simulink model "Copy_of_NolinearPMP"  (R2019b)
settings: Solver=ode14x  StartTime=0.0  StopTime=t_cyc(end)  FixedStep=0.01  RelTol=1e-3  EnableMultiTasking=on
values from neighbouring files (symbols this model uses):
  alph_cyc = [0 0 0 0 0 0 0 0 0 0 0 0 ... (6685 elements, 6685x1)]    [SUMOInfo.mat]
  distance_edge = [989.64 2422.29 340.79 475.79 617.54 348 731.29 242.71 400.49 162.3 1072.99 342.19 ... (42 elements, 42x1)]    [SUMOInfo.mat]    (also in msfun_EMS_PMP.m = block.DialogPrm(15).Data)
  ess_ro = block.DialogPrm(9).Data    [msfun_EMS_PMP.m]
  ess_soc = block.DialogPrm(7).Data    [msfun_EMS_PMP.m]
  ess_voc = block.DialogPrm(8).Data    [msfun_EMS_PMP.m]
  K = block.DialogPrm(12).Data    [msfun_EMS_PMP.m]
  meangrade = zeros(42,1)    [data_load.m]
  Np = block.DialogPrm(11).Data    [msfun_EMS_PMP.m]
  Ns = block.DialogPrm(10).Data    [msfun_EMS_PMP.m]
  p2 = block.DialogPrm(13).Data    [msfun_EMS_PMP.m]
  PM = block.DialogPrm(4).Data    [msfun_EMS_PMP.m]
  Qnom = block.DialogPrm(5).Data    [msfun_EMS_PMP.m]
  ratio = block.DialogPrm(3).Data    [msfun_EMS_PMP.m]
  regR = zeros(42,1)    [data_load.m]    (also in msfun_EMS_PMP.m = block.DialogPrm(6).Data)
  s = [0 1.19972903225 3.59869534029 7.19334975441 11.9718409783 17.9064273504 24.9452359727 33.006043999 41.9755365162 51.7163644674 62.0808345859 72.9273231974 ... (6685 elements, 6685x1)]    [SUMOInfo.mat]
  t_cyc = [1 2 3 4 5 6 7 8 9 10 11 12 ... (6685 elements, 6685x1)]    [SUMOInfo.mat]
  trafficspeed = block.DialogPrm(1).Data    [msfun_EMS_PMP.m]
  v_cyc = [0 4.31902451611 8.63627870893 12.9407558908 17.202568406 21.3645109397 25.3397110401 29.0189088948 32.2901730621 35.0669806241 37.3120924268 39.0473590013 ... (6685 elements, 6685x1)]    [SUMOInfo.mat]
undefined symbols (not defined in the file or in its folder): A_wind, Cd, Ce, delta1, delta2, eff_m, fuelrate, i0, Je, Jg, ki, kp, lambda_f, Ld, Lq, MaxFuelRate, meanspeed_record, motor_nt, nOpt, p, Pdmd_distribution, PgOpt, Qmax, R, r_wh, segmentID, Ta, veh_mass, x0
libraries: simulink x4, dsparch4 x1
settings Model: SimulationMode=accelerator  Creator=chenyaoqi  LastModifiedBy=Administrator
settings SolverCC: NumberNewtonIterations=2
settings DataIOCC: ReturnWorkspaceOutputs=off
settings OptimizationCC: LifeSpan=inf
settings DebuggingCC: SFUnexpectedBacktrackingDiag=warning  SFNoUnconditionalDefaultTransitionDiag=warning  ArithmeticOperatorsInVariantConditions=warning
settings SFSimCC: SimUseLocalCustomCode=off  CustomCodeUndefinedFunction=UseInterfaceOnly
settings RTWCC: RTWUseLocalCustomCode=off
settings CodeAppCC: StateflowObjectComments=on
settings GRTTargetCC: TargetLangStandard=C89/C90 (ANSI)  GeneratePreprocessorConditionals=Disable all
settings ConfigComp: CovMetricSettings=dw  CovHtmlReporting=on  CovSaveCumulativeToWorkspaceVar=on  CovSaveSingleToWorkspaceVar=on  CovExternalEMLEnable=off

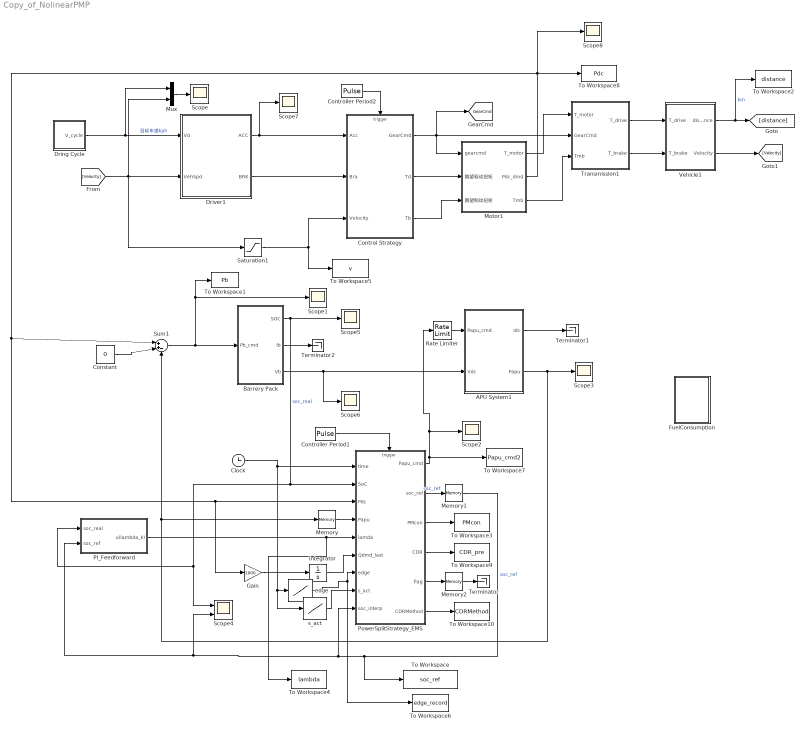
== system Copy_of_NolinearPMP ==
  APU System1 : Subsystem
  Barrery Pack : Subsystem
  Clock : Clock
  Constant : Constant  Value=0
  Control Strategy : Stateflow chart  TreatAsAtomicUnit=on
  Controller Period1 : DiscretePulseGenerator  PulseType=Time based  Period=1  PulseWidth=50
  Controller Period2 : DiscretePulseGenerator  PulseType=Time based  Period=0.1  PulseWidth=10
  Dring Cycle : Subsystem
  Driver1 : Subsystem
  FuelConsumption : Subsystem
  Gain : Gain  Gain=1000
  Integrator : Integrator
  Memory : Memory
  Memory1 : Memory
  Memory2 : Memory  InheritSampleTime=on
  Motor1 : Subsystem
  Mux : Mux  Inputs=2
  PI_Feedforward : Subsystem
  PowerSplitStrategy_EMS : Subsystem
  Rate Limiter : RateLimiter  RisingSlewLimit=8  FallingSlewLimit=-10
  Saturation1 : Saturate  UpperLimit=200  LowerLimit=0
  Scope{,1..3,5..8} (8 alike) : Scope
  Scope4 : Scope  NumInputPorts=2
  Sum1 : Sum  Inputs=|++-
  Terminator : Terminator
  Terminator1 : Terminator
  Terminator2 : Terminator
  To Workspace : ToWorkspace  VariableName=soc_ref  SampleTime=-1
  To Workspace1 : ToWorkspace  VariableName=Pb  SampleTime=-1
  To Workspace10 : ToWorkspace  VariableName=CDRMethod  SampleTime=-1
  To Workspace2 : ToWorkspace  VariableName=distance  SampleTime=-1
  To Workspace3 : ToWorkspace  VariableName=PMcon  SampleTime=-1
  To Workspace4 : ToWorkspace  VariableName=lambda  SampleTime=-1
  To Workspace5 : ToWorkspace  VariableName=v  SampleTime=-1
  To Workspace6 : ToWorkspace  VariableName=edge_record  SampleTime=-1
  To Workspace7 : ToWorkspace  VariableName=Papu_cmd2  SampleTime=-1
  To Workspace8 : ToWorkspace  VariableName=Pdc  SampleTime=-1
  To Workspace9 : ToWorkspace  VariableName=CDR_pre  SampleTime=-1
  Transmission1 : Subsystem
  Vehicle1 : Subsystem
  edge : Lookup  InputValues=t_cyc  Table=segmentID  LookUpMeth=Use Input Nearest
  s_act : Lookup  InputValues=t_cyc  Table=s
  tag scope: GearCmd=global
  wires:
  Barrery Pack/2(Ib) -> Terminator2/1
  Constant/1 -> Sum1/2
  PowerSplitStrategy_EMS/1(Papu_cmd) -> To Workspace7/1, Rate Limiter/1, Scope2/1
  Sum1/1 -> Barrery Pack/1(Pb_cmd), To Workspace1/1, Scope1/1
  APU System1/1(Idc) -> Terminator1/1
  Barrery Pack/3(Vb) -> Scope6/1, APU System1/2(Vdc)
  Rate Limiter/1 -> APU System1/1(Papu_cmd)
  Dring Cycle/1(V_cycle) -> Driver1/1(Vd), Mux/1  "目标车速kph"
  [Velocity] -> Driver1/2(VehSpd), Mux/2, Saturation1/1
  Saturation1/1 -> Control Strategy/3(Velocity), To Workspace5/1
  Barrery Pack/1(SOC) -> Scope5/1, Scope4/1, PI_Feedforward/1(soc_real), PowerSplitStrategy_EMS/2(SoC)  "soc_real"
  APU System1/2(Papu) -> Scope3/1, Sum1/3, Memory/1
  Controller Period1/1 -> PowerSplitStrategy_EMS/Trigger
  Mux/1 -> Scope/1
  Transmission1/1(T_drive) -> Vehicle1/1(T_drive)
  Motor1/1(T_motor) -> Transmission1/1(T_motor)
  Motor1/2(Pdc_dmd) -> Scope8/1, To Workspace8/1, Sum1/1, Gain/1, PowerSplitStrategy_EMS/3(Pdc)
  Controller Period2/1 -> Control Strategy/Trigger
  Control Strategy/1(GearCmd) -> [GearCmd], Transmission1/2(GearCmd), Motor1/1(gearcmd)
  Vehicle1/1(distance) -> [distance], To Workspace2/1  "km"
  Vehicle1/2(Velocity) -> [Velocity]
  Motor1/3(Tmb) -> Transmission1/3(Tmb)
  Control Strategy/2(Td) -> Motor1/2(期望驱动扭矩)
  Control Strategy/3(Tb) -> Motor1/3(期望制动扭矩)
  Transmission1/2(T_brake) -> Vehicle1/2(T_brake)
  Driver1/1(ACC) -> Scope7/1, Control Strategy/1(Acc)
  Driver1/2(BRK) -> Control Strategy/2(Bra)
  Memory/1 -> PowerSplitStrategy_EMS/4(Papu)
  Integrator/1 -> PowerSplitStrategy_EMS/6(Qdmd_last)
  edge/1 -> To Workspace6/1, PowerSplitStrategy_EMS/7(edge)
  Clock/1 -> PowerSplitStrategy_EMS/1(time), s_act/1, edge/1
  s_act/1 -> PowerSplitStrategy_EMS/8(s_act)
  Gain/1 -> Integrator/1
  Memory1/1 -> PI_Feedforward/2(soc_ref), Scope4/2, PowerSplitStrategy_EMS/9(soc_interp), To Workspace/1  "soc_ref"
  PowerSplitStrategy_EMS/3(PMcon) -> To Workspace3/1
  PowerSplitStrategy_EMS/4(CDR) -> To Workspace9/1
  PowerSplitStrategy_EMS/5(flag) -> Memory2/1
  Memory2/1 -> Terminator/1
  PowerSplitStrategy_EMS/6(CDRMethod) -> To Workspace10/1
  PI_Feedforward/1(u(lambda_k)) -> To Workspace4/1, PowerSplitStrategy_EMS/5(lamda)
  PowerSplitStrategy_EMS/2(soc_ref) -> Memory1/1  "soc_ref"

== system Copy_of_NolinearPMP/APU System1 ==
  Papu_cmd : Inport
  Vdc : Inport  Port=2
  "APU Optimal Operating LIne2 " : Lookup_n-D  NumberOfTableDimensions=1  BreakpointsForDimension1=PgOpt  Table=nOpt  InputSameDT=on
  Divide1 : Product  Inputs=/*
  Gain : Gain  Gain=9549
  Genset : Subsystem
  To Workspace1 : ToWorkspace  VariableName=Papu  SampleTime=-1
  Idc : Outport
  Papu : Outport  Port=2
  tag scope: Papu=global
  wires:
  Papu_cmd/1 -> Gain/1, "APU Optimal Operating LIne2 "/1
  Gain/1 -> Divide1/2
  Genset/1(Ig) -> Idc/1
  Genset/2(Papu) -> To Workspace1/1, Papu/1, [Papu]
  Vdc/1 -> Genset/2(Vdc)  "pack电压"
  "APU Optimal Operating LIne2 "/1 -> Divide1/1, Genset/3(omega_cmd)  "期望转速rpm"
  Divide1/1 -> Genset/1(T_cmd)  "期望扭矩"

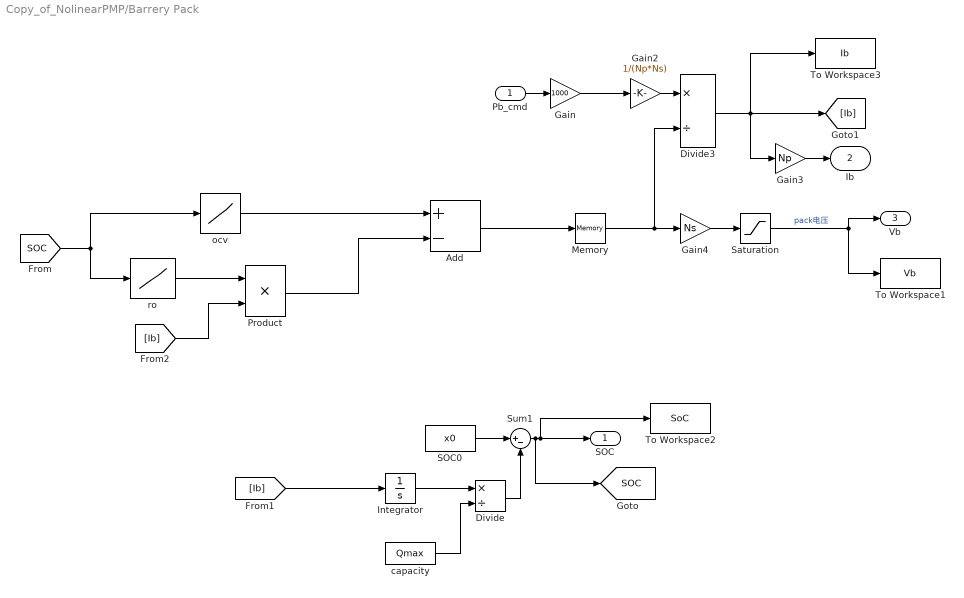
== system Copy_of_NolinearPMP/Barrery Pack ==
  Pb_cmd : Inport
  Add : Sum  Inputs=+-
  Divide : Product  Inputs=*/
  Divide3 : Product  Inputs=*/
  Gain : Gain  Gain=1000
  Gain2 : Gain  Gain=1/(Np*Ns)
  Gain3 : Gain  Gain=Np
  Gain4 : Gain  Gain=Ns
  Integrator : Integrator
  Memory : Memory  InitialCondition=4
  Product : Product
  SOC0 : Constant  Value=x0
  Saturation : Saturate  UpperLimit=453.6  LowerLimit=302.4
  Sum1 : Sum  Inputs=|+-
  To Workspace1 : ToWorkspace  VariableName=Vb  SampleTime=-1
  To Workspace2 : ToWorkspace  VariableName=SoC  SampleTime=-1
  To Workspace3 : ToWorkspace  VariableName=Ib  SampleTime=-1
  capacity : Constant  Value=Qmax
  ocv : Lookup_n-D  NumberOfTableDimensions=1  BreakpointsForDimension1=ess_soc  Table=ess_voc  InternalRulePriority=Speed  RndMeth=Simplest  InputSameDT=on
  ro : Lookup_n-D  NumberOfTableDimensions=1  BreakpointsForDimension1=ess_soc  Table=ess_ro  InternalRulePriority=Speed  RndMeth=Simplest  InputSameDT=on
  SOC : Outport
  Ib : Outport  Port=2
  Vb : Outport  Port=3
  tag scope: SOC=global
  wires:
  capacity/1 -> Divide/2
  Divide/1 -> Sum1/2
  SOC0/1 -> Sum1/1
  Sum1/1 -> [SOC], SOC/1, To Workspace2/1
  Integrator/1 -> Divide/1
  Pb_cmd/1 -> Gain/1
  Gain/1 -> Gain2/1
  Divide3/1 -> To Workspace3/1, Gain3/1, [Ib]
  Memory/1 -> Divide3/2, Gain4/1
  Gain2/1 -> Divide3/1
  [SOC] -> ocv/1, ro/1
  Gain3/1 -> Ib/1
  Gain4/1 -> Saturation/1
  Saturation/1 -> To Workspace1/1, Vb/1  "pack电压"
  ro/1 -> Product/1
  [Ib] -> Product/2
  Add/1 -> Memory/1
  ocv/1 -> Add/1
  Product/1 -> Add/2
  [Ib] -> Integrator/1

== system Copy_of_NolinearPMP/Dring Cycle ==
  Clock : Clock
  To Workspace1 : ToWorkspace  VariableName=time  SampleTime=-1
  cyc : Lookup  InputValues=t_cyc  Table=v_cyc  LookUpMeth=Interpolation-Use End Values
  V_cycle : Outport
  wires:
  Clock/1 -> cyc/1, To Workspace1/1
  cyc/1 -> V_cycle/1  "kph"

== system Copy_of_NolinearPMP/Driver1 ==
  Vd : Inport
  VehSpd : Inport  Port=2
  Clock : Clock
  Driver : Subsystem
  Mux1 : Mux  Inputs=2
  alph_cyc : Lookup  InputValues=t_cyc  Table=alph_cyc
  黄色-模型车速、蓝色-实际车速 : Scope
  ACC : Outport
  BRK : Outport  Port=2
  wires:
  VehSpd/1 -> Driver/2(VelFdbk), Mux1/2  "模型仿真车速"
  Vd/1 -> Mux1/1, Driver/1(VelRef)
  Mux1/1 -> 黄色-模型车速、蓝色-实际车速/1
  Driver/1(AccelCmd) -> ACC/1
  Driver/2(BrkCmd) -> BRK/1
  alph_cyc/1 -> Driver/3(Grade)
  Clock/1 -> alph_cyc/1

== system Copy_of_NolinearPMP/FuelConsumption ==
  Constant : Constant  Value=0
  FuelRate : Fcn  Expr=Ce(1)+Ce(2)*u(1)+Ce(3)*u(2)+Ce(4)*u(1)*u(1)+Ce(5)*u(1)*u(2)+Ce(6)*u(2)*u(2)+Ce(7)*u(1)*u(1)*u(1)+Ce(8)*u(1)*u(1)*u(2)+Ce(9)*u(1)*u(2)*u(2)+Ce(10)*u(2)*u(2)*u(2)
  Gain : Gain  Gain=30/pi
  Integrator : Integrator
  Mux : Mux  Inputs=2
  Switch : Switch
  To Workspace : ToWorkspace  VariableName=CumulativeFC  SampleTime=-1
  To Workspace1 : ToWorkspace  VariableName=FC_instant  SampleTime=-1
  wires:
  [Te] -> Mux/2
  Mux/1 -> FuelRate/1
  [omega_e] -> Gain/1
  Gain/1 -> Mux/1  "rpm"
  Integrator/1 -> To Workspace/1
  FuelRate/1 -> Switch/2, Switch/1
  Switch/1 -> Integrator/1, To Workspace1/1
  Constant/1 -> Switch/3

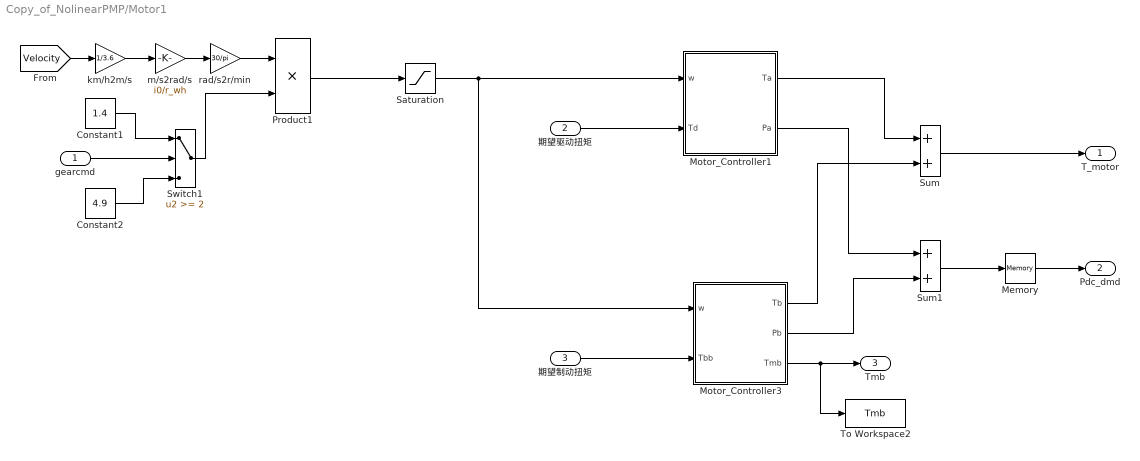
== system Copy_of_NolinearPMP/Motor1 ==
  gearcmd : Inport
  期望驱动扭矩 : Inport  Port=2
  期望制动扭矩 : Inport  Port=3
  Constant1 : Constant  Value=1.4
  Constant2 : Constant  Value=4.9
  Memory : Memory  InheritSampleTime=on
  Motor_Controller1 : Subsystem
  Motor_Controller3 : Subsystem
  Product1 : Product  RndMeth=Zero
  Saturation : Saturate  UpperLimit=4200  LowerLimit=0  ZeroCross=off
  Sum : Sum
  Sum1 : Sum
  Switch1 : Switch  Threshold=2  ZeroCross=off
  To Workspace2 : ToWorkspace  VariableName=Tmb  SampleTime=-1
      settings: Decimation=100
  km/h2m/s : Gain  Gain=1/3.6
  m/s2rad/s : Gain  Gain=i0/r_wh
  rad/s2r/min : Gain  Gain=30/pi
  T_motor : Outport
  Pdc_dmd : Outport  Port=2
  Tmb : Outport  Port=3
  wires:
  Sum1/1 -> Memory/1
  km/h2m/s/1 -> m/s2rad/s/1
  [Velocity] -> km/h2m/s/1
  gearcmd/1 -> Switch1/2
  Constant1/1 -> Switch1/1
  Constant2/1 -> Switch1/3
  Switch1/1 -> Product1/2
  Sum/1 -> T_motor/1
  m/s2rad/s/1 -> rad/s2r/min/1
  rad/s2r/min/1 -> Product1/1
  Product1/1 -> Saturation/1
  Memory/1 -> Pdc_dmd/1
  Saturation/1 -> Motor_Controller1/1(w), Motor_Controller3/1(w)
  期望驱动扭矩/1 -> Motor_Controller1/2(Td)
  期望制动扭矩/1 -> Motor_Controller3/2(Tbb)
  Motor_Controller3/3(Tmb) -> To Workspace2/1, Tmb/1
  Motor_Controller3/2(Pb) -> Sum1/2
  Motor_Controller1/2(Pa) -> Sum1/1
  Motor_Controller1/1(Ta) -> Sum/1
  Motor_Controller3/1(Tb) -> Sum/2

== system Copy_of_NolinearPMP/PI_Feedforward ==
  soc_real : Inport
  soc_ref : Inport  Port=2
  Add : Sum  Inputs=+-
  Analog Filter Design : dsparch4/Analog Filter Design  Commented=on  method=Butterworth  filttype=Lowpass  N=1  Wlo=0.5  Whi=80  Rp=2  Rs=40
  PID Controller : simulink/Continuous/PID Controller  Controller=PI  Form=Parallel  TimeDomain=Continuous-time  SampleTime=-1  IntegratorMethod=Forward Euler  FilterMethod=Forward Euler  ControllerParametersSource=internal  P=kp  I=ki  D=0  UseFilter=on  N=100  TunerSelectOption=Transfer Function Based (PID Tuner App)  InitialConditionSource=internal  InitialConditionForIntegrator=-13066.5  InitialConditionForFilter=0  DifferentiatorICPrevScaledInput=0  ExternalReset=none  TrackingMode=off  Kt=1  LimitOutput=off  UpperSaturationLimit=inf  LowerSaturationLimit=-inf  LinearizeAsGain=on  AntiWindupMode=none  Kb=1  POutMin=[]  POutMax=[]  IOutMin=[]  IOutMax=[]  DOutMin=[]  DOutMax=[]  NOutMin=[]  NOutMax=[]  SumOutMin=[]  SumOutMax=[]  SaturationOutMin=[]  SaturationOutMax=[]  PParamMin=[]  PParamMax=[]  IParamMin=[]  IParamMax=[]  DParamMin=[]  DParamMax=[]  NParamMin=[]  NParamMax=[]  KbParamMin=[]  KbParamMax=[]  KtParamMin=[]  KtParamMax=[]  KbOutMin=[]  KbOutMax=[]  KtOutMin=[]  KtOutMax=[]  IntegratorOutMin=[]  IntegratorOutMax=[]  FilterOutMin=[]  FilterOutMax=[]  SumI1OutMin=[]  SumI1OutMax=[]  SumI2OutMin=[]  SumI2OutMax=[]  SumI3OutMin=[]  SumI3OutMax=[]  SumI4OutMin=[]  SumI4OutMax=[]  SumDOutMin=[]  SumDOutMax=[]  DifferentiatorOutMin=[]  DifferentiatorOutMax=[]  FilterDiffOutCoefMin=[]  FilterDiffOutCoefMax=[]  ReciprocalOutMin=[]  ReciprocalOutMax=[]  SumDenOutMin=[]  SumDenOutMax=[]  SumNumOutMin=[]  SumNumOutMax=[]  DivideOutMin=[]  DivideOutMax=[]  IntegratorContinuousStateAttributes=''  IntegratorStateMustResolveToSignalObject=off  IntegratorRTWStateStorageClass=Auto  FilterContinuousStateAttributes=''  FilterStateMustResolveToSignalObject=off  FilterRTWStateStorageClass=Auto  ParallelPVariant=InternalParameters  IdealPVariant=Disabled  IVariant=InternalParameters  DVariant=Disabled  IntegratorVariant=Continuous  SatVariant=Disabled  AWVariant=Passthrough  PCopyVariant=Disabled  TRVariant=Disabled  FdbkBlocksVariant=Forward  IdealPFdbkVariant=Disabled  SatFdbkVariant=Disabled  DerivativeFilterVariant=Disabled  NVariant=Disabled  NCopyVariant=Disabled_SignalSpec  FilterICVariant=Disabled  IntegratorICVariant=InternalICs  ExternalResetVariant=Disabled  TRSumVariant=Passthrough  SumFdbkVariant=Disabled  SumVariant=Sum_PI
  u(lambda_k) : Outport  InitialOutput=-13060  VectorParamsAs1DForOutWhenUnconnected=off
  wires:
  soc_real/1 -> Add/1
  soc_ref/1 -> Add/2
  PID Controller/1 -> u(lambda_k)/1  "delta_u"
  Add/1 -> PID Controller/1  "e(k)"

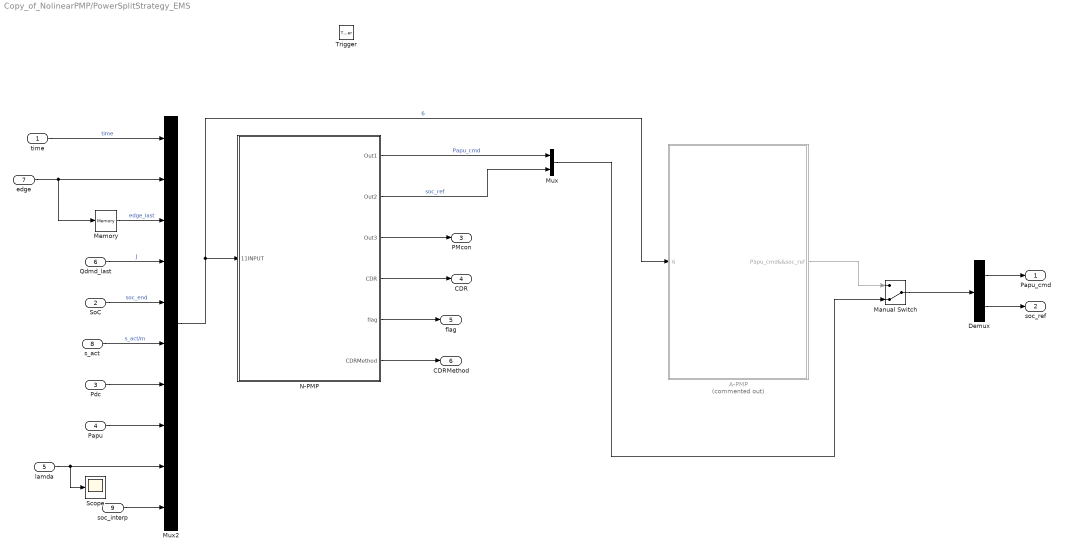
== system Copy_of_NolinearPMP/PowerSplitStrategy_EMS ==
  time : Inport
  SoC : Inport  Port=2
  Pdc : Inport  Port=3
  Papu : Inport  Port=4
  lamda : Inport  Port=5
  Qdmd_last : Inport  Port=6
  edge : Inport  Port=7
  s_act : Inport  Port=8
  soc_interp : Inport  Port=9
  Trigger : TriggerPort  VariantControl=Variant  PortDimensions=1
  A-PMP : Subsystem  Commented=on
  Demux : Demux  Outputs=2
  Manual Switch : ManualSwitch  CurrentSetting=0
  Memory : Memory  InitialCondition=1  InheritSampleTime=on
  Mux : Mux  Inputs=2
  Mux2 : Mux  Inputs=10
  N-PMP : Subsystem
  Scope : Scope
  Papu_cmd : Outport
  soc_ref : Outport  Port=2
  PMcon : Outport  Port=3  VectorParamsAs1DForOutWhenUnconnected=off
  CDR : Outport  Port=4  VectorParamsAs1DForOutWhenUnconnected=off
  flag : Outport  Port=5  VectorParamsAs1DForOutWhenUnconnected=off
  CDRMethod : Outport  Port=6  VectorParamsAs1DForOutWhenUnconnected=off
  wires:
  Mux2/1 -> A-PMP/1(6), N-PMP/1(11INPUT)  "6"
  A-PMP/1(Papu_cmd&&soc_ref) -> Manual Switch/1
  Mux/1 -> Manual Switch/2
  Manual Switch/1 -> Demux/1
  Demux/1 -> Papu_cmd/1
  Demux/2 -> soc_ref/1
  lamda/1 -> Scope/1, Mux2/9
  N-PMP/1(Out1) -> Mux/1  "Papu_cmd"
  N-PMP/2(Out2) -> Mux/2  "soc_ref"
  time/1 -> Mux2/1  "time"
  edge/1 -> Mux2/2, Memory/1
  Memory/1 -> Mux2/3  "edge_last"
  Pdc/1 -> Mux2/7
  SoC/1 -> Mux2/5  "soc_end"
  s_act/1 -> Mux2/6  "s_act/m"
  Papu/1 -> Mux2/8
  Qdmd_last/1 -> Mux2/4  "J"
  N-PMP/3(Out3) -> PMcon/1
  N-PMP/4(CDR) -> CDR/1
  soc_interp/1 -> Mux2/10
  N-PMP/5(flag) -> flag/1
  N-PMP/6(CDRMethod) -> CDRMethod/1

== system Copy_of_NolinearPMP/Transmission1 ==
  T_motor : Inport
  GearCmd : Inport  Port=2
  Tmb : Inport  Port=3
  Gain : Gain  Gain=0.95
  Gain1 : Gain  Gain=0.95
  Lookup Table : Lookup  InputValues=[1,2]  Table=[4.9,1.4]
  Product : Product  RndMeth=Zero
  Product1 : Product  RndMeth=Zero
  T_drive : Outport
  T_brake : Outport  Port=2
  wires:
  GearCmd/1 -> Lookup Table/1
  T_motor/1 -> Product/1
  Lookup Table/1 -> Product/2, Product1/2
  Gain/1 -> T_drive/1
  Product/1 -> Gain/1
  Tmb/1 -> Product1/1
  Gain1/1 -> T_brake/1
  Product1/1 -> Gain1/1

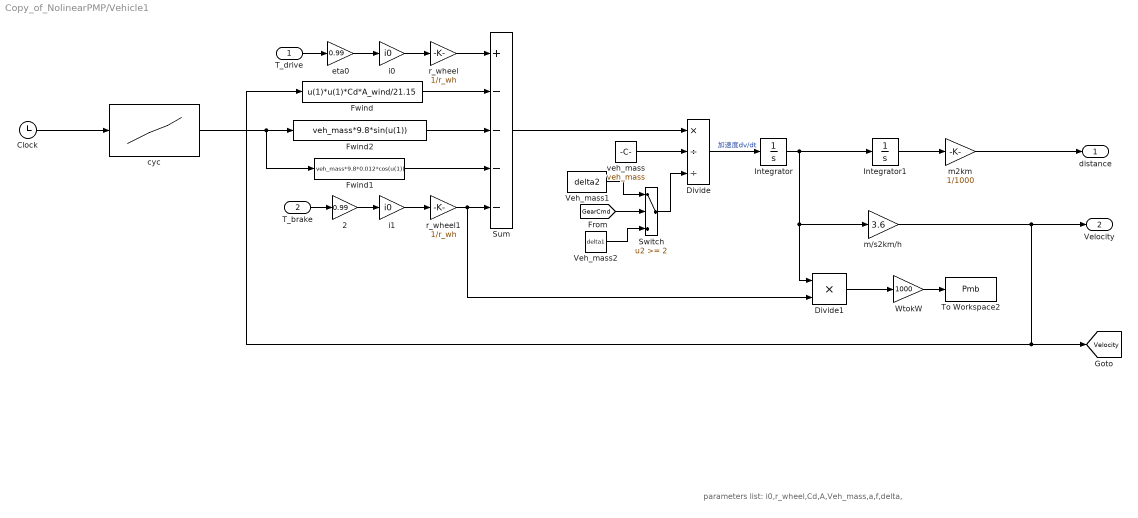
== system Copy_of_NolinearPMP/Vehicle1 ==
  note: parameters list: i0,r_wheel,Cd,A,Veh_mass,a,f,delta,
  T_drive : Inport
  T_brake : Inport  Port=2
  2 : Gain  Gain=0.99
  Clock : Clock
  Divide : Product  Inputs=*//
  Divide1 : Product  Inputs=**
  Fwind : Fcn  Expr=u(1)*u(1)*Cd*A_wind/21.15
  Fwind1 : Fcn  Expr=veh_mass*9.8*0.012*cos(u(1))
  Fwind2 : Fcn  Expr=veh_mass*9.8*sin(u(1))
  Integrator : Integrator  LimitOutput=on  UpperSaturationLimit=100  LowerSaturationLimit=0
  Integrator1 : Integrator
  Sum : Sum  Inputs=+----
  Switch : Switch  Threshold=2  ZeroCross=off
  To Workspace2 : ToWorkspace  VariableName=Pmb  SampleTime=-1
  Veh_mass1 : Constant  Value=delta2
  Veh_mass2 : Constant  Value=delta1
  WtokW : Gain  Gain=1000
  cyc : Lookup  InputValues=t_cyc  Table=alph_cyc
  eta0 : Gain  Gain=0.99
  i0 : Gain  Gain=i0
  i1 : Gain  Gain=i0
  m/s2km/h : Gain  Gain=3.6
  m2km : Gain  Gain=1/1000
  r_wheel : Gain  Gain=1/r_wh
  r_wheel1 : Gain  Gain=1/r_wh
  veh_mass : Constant  Value=veh_mass
  distance : Outport
  Velocity : Outport  Port=2
  tag scope: Velocity=global
  wires:
  Fwind1/1 -> Sum/4
  Fwind2/1 -> Sum/3
  Fwind/1 -> Sum/2
  r_wheel/1 -> Sum/1
  Sum/1 -> Divide/1
  veh_mass/1 -> Divide/2
  Divide/1 -> Integrator/1  "加速度dv/dt"
  Integrator/1 -> Divide1/1, m/s2km/h/1, Integrator1/1
  m/s2km/h/1 -> Velocity/1, Fwind/1, [Velocity]
  Integrator1/1 -> m2km/1
  m2km/1 -> distance/1
  Switch/1 -> Divide/3
  Veh_mass1/1 -> Switch/1
  [GearCmd] -> Switch/2
  Veh_mass2/1 -> Switch/3
  cyc/1 -> Fwind1/1, Fwind2/1
  Clock/1 -> cyc/1
  i1/1 -> r_wheel1/1
  T_brake/1 -> 2/1
  2/1 -> i1/1
  r_wheel1/1 -> Divide1/2, Sum/5
  Divide1/1 -> WtokW/1
  WtokW/1 -> To Workspace2/1
  T_drive/1 -> eta0/1
  eta0/1 -> i0/1
  i0/1 -> r_wheel/1

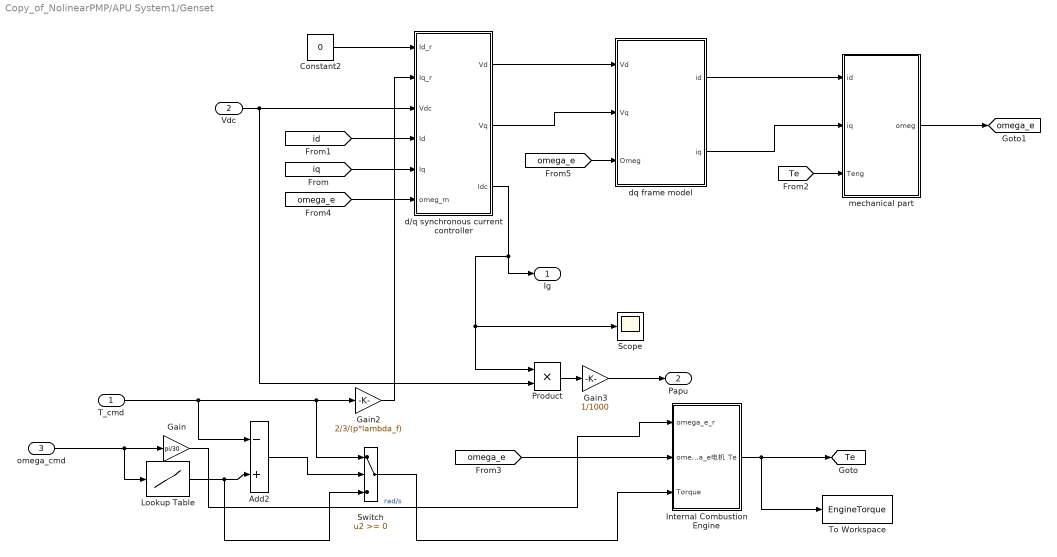
== system Copy_of_NolinearPMP/APU System1/Genset ==
  T_cmd : Inport
  Vdc : Inport  Port=2
  omega_cmd : Inport  Port=3
  Add2 : Sum  Inputs=-+
  Constant2 : Constant  Value=0
  Gain : Gain  Gain=pi/30
  Gain2 : Gain  Gain=2/3/(p*lambda_f)
  Gain3 : Gain  Gain=1/1000
  Internal Combustion Engine : Subsystem
  Lookup Table : Lookup  InputValues=[850,1000,1250,1500,1750,2000,2250,2500,2750,3000,3250,3500,3750,4000]  Table=[195,195,195,195.9,244.1,270.2,272.7,269.1,266.6,261.5,257.7,242.9,229.9,221.4]
  Product : Product  RndMeth=Zero
  Scope : Scope
  Switch : Switch
  To Workspace : ToWorkspace  VariableName=EngineTorque  SampleTime=-1
  d/q synchronous current controller : Subsystem
  "dq frame model " : Subsystem
  mechanical part : Subsystem
  Ig : Outport
  Papu : Outport  Port=2
  tag scope: Te=global, omega_e=global
  wires:
  mechanical part/1(omeg) -> [omega_e]
  "dq frame model "/1(id) -> mechanical part/1(id)
  "dq frame model "/2(iq) -> mechanical part/2(iq)
  [Te] -> mechanical part/3(Teng)
  [id] -> d/q synchronous current controller/4(Id)
  [iq] -> d/q synchronous current controller/5(Iq)
  [omega_e] -> Internal Combustion Engine/2(omega_e电机)
  [omega_e] -> d/q synchronous current controller/6(omeg_m)
  [omega_e] -> "dq frame model "/3(Omeg)
  Constant2/1 -> d/q synchronous current controller/1(Id_r)
  Vdc/1 -> Product/2, d/q synchronous current controller/3(Vdc)
  d/q synchronous current controller/3(Idc) -> Scope/1, Product/1, Ig/1
  Product/1 -> Gain3/1
  Internal Combustion Engine/1(Te) -> [Te], To Workspace/1
  omega_cmd/1 -> Lookup Table/1, Gain/1
  Gain2/1 -> d/q synchronous current controller/2(Iq_r)
  d/q synchronous current controller/1(Vd) -> "dq frame model "/1(Vd)
  d/q synchronous current controller/2(Vq) -> "dq frame model "/2(Vq)
  T_cmd/1 -> Add2/1, Gain2/1, Switch/1
  Lookup Table/1 -> Add2/2, Switch/3
  Add2/1 -> Switch/2
  Switch/1 -> Internal Combustion Engine/3(Torque)
  Gain/1 -> Internal Combustion Engine/1(omega_e_r)  "rad/s"
  Gain3/1 -> Papu/1

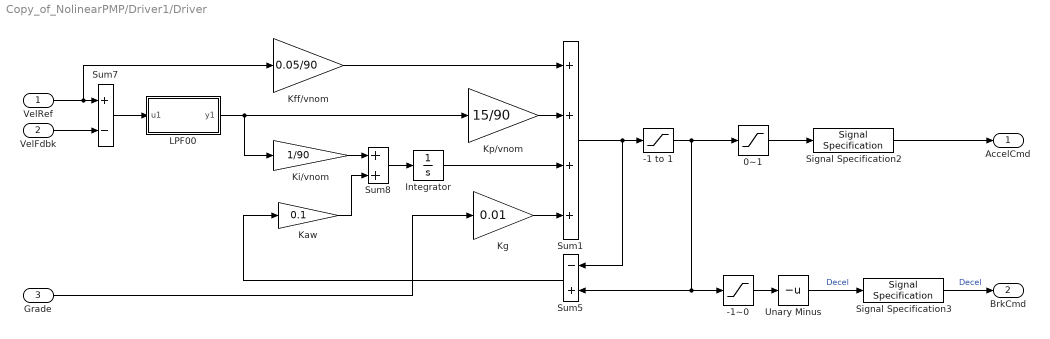
== system Copy_of_NolinearPMP/Driver1/Driver ==
  VelRef : Inport
  VelFdbk : Inport  Port=2
  Grade : Inport  Port=3
  "-1 to 1 " : Saturate  UpperLimit=1  LowerLimit=-1
  -1~0 : Saturate  UpperLimit=0  LowerLimit=-1  ZeroCross=off
  0~1 : Saturate  UpperLimit=1  LowerLimit=0  ZeroCross=off
  Integrator : Integrator  LimitOutput=on  UpperSaturationLimit=1  LowerSaturationLimit=-1
  Kaw : Gain  Gain=0.1  SaturateOnIntegerOverflow=on  OutDataTypeStr=Inherit: Same as input  ParamDataTypeStr=Inherit: Same as input
  Kff/vnom : Gain  Gain=0.05/90  SaturateOnIntegerOverflow=on  OutDataTypeStr=Inherit: Same as input  ParamDataTypeStr=Inherit: Same as input
  Kg : Gain  Gain=0.01  SaturateOnIntegerOverflow=on  OutDataTypeStr=Inherit: Same as input  ParamDataTypeStr=Inherit: Same as input
  Ki/vnom : Gain  Gain=1/90  SaturateOnIntegerOverflow=on  OutDataTypeStr=Inherit: Same as input  ParamDataTypeStr=Inherit: Same as input
  Kp/vnom : Gain  Gain=15/90  SaturateOnIntegerOverflow=on  OutDataTypeStr=Inherit: Same as input  ParamDataTypeStr=Inherit: Same as input
  LPF00 : Subsystem
  Signal Specification2 : SignalSpecification
  Signal Specification3 : SignalSpecification
  Sum1 : Sum  Inputs=++++  SaturateOnIntegerOverflow=on  InputSameDT=on  OutDataTypeStr=Inherit: Same as first input
  Sum5 : Sum  Inputs=-+  SaturateOnIntegerOverflow=on  InputSameDT=on  OutDataTypeStr=Inherit: Same as first input
  Sum7 : Sum  Inputs=+-  SaturateOnIntegerOverflow=on  InputSameDT=on  OutDataTypeStr=Inherit: Same as first input
  Sum8 : Sum  SaturateOnIntegerOverflow=on  InputSameDT=on  OutDataTypeStr=Inherit: Same as first input
  Unary Minus : UnaryMinus
  AccelCmd : Outport  InitialOutput=0
  BrkCmd : Outport  Port=2  InitialOutput=0
  wires:
  Sum7/1 -> LPF00/1(u1)
  0~1/1 -> Signal Specification2/1
  Sum1/1 -> "-1 to 1 "/1, Sum5/1
  LPF00/1(y1) -> Kp/vnom/1, Ki/vnom/1
  -1~0/1 -> Unary Minus/1
  VelFdbk/1 -> Sum7/2
  Kg/1 -> Sum1/4
  Grade/1 -> Kg/1
  Sum8/1 -> Integrator/1
  Kaw/1 -> Sum8/2
  Kp/vnom/1 -> Sum1/2
  "-1 to 1 "/1 -> 0~1/1, -1~0/1, Sum5/2
  VelRef/1 -> Sum7/1, Kff/vnom/1
  Unary Minus/1 -> Signal Specification3/1  "Decel"
  Kff/vnom/1 -> Sum1/1
  Integrator/1 -> Sum1/3
  Sum5/1 -> Kaw/1
  Ki/vnom/1 -> Sum8/1
  Signal Specification3/1 -> BrkCmd/1  "Decel"
  Signal Specification2/1 -> AccelCmd/1

== system Copy_of_NolinearPMP/Motor1/Motor_Controller1 ==
  w : Inport
  Td : Inport  Port=2
  2-D Lookup Table : Lookup_n-D  BreakpointsForDimension1=0:500:4500  BreakpointsForDimension2=-850:50:850  Table=eff_m  InternalRulePriority=Speed  RndMeth=Simplest  InputSameDT=on
  Divide : Product  Inputs=*/
  Gain2 : Gain  Gain=1/9549
  Gain3 : Gain
  Lookup Table (3-D) : Lookup_n-D  BreakpointsForDimension1=[500,1000,1500,2000,2500,3000,3500,4000,4200]  BreakpointsForDimension2=[0,800,1600,2400,3200,4000,4800,5600,6400,7200,8000]  BreakpointsForDimension3=[425,445]  Table=Ta  InputSameDT=on
  Product : Product  RndMeth=Zero
  Saturation : Saturate  UpperLimit=1  LowerLimit=0.1
  Ta : Outport
  Pa : Outport  Port=2
  wires:
  Divide/1 -> Pa/1
  Td/1 -> Lookup Table (3-D)/2
  Lookup Table (3-D)/1 -> Product/1, Gain3/1
  Product/1 -> Gain2/1
  w/1 -> Lookup Table (3-D)/1, Product/2, 2-D Lookup Table/1
  Saturation/1 -> Divide/2
  2-D Lookup Table/1 -> Saturation/1
  Gain2/1 -> Divide/1
  Gain3/1 -> 2-D Lookup Table/2, Ta/1

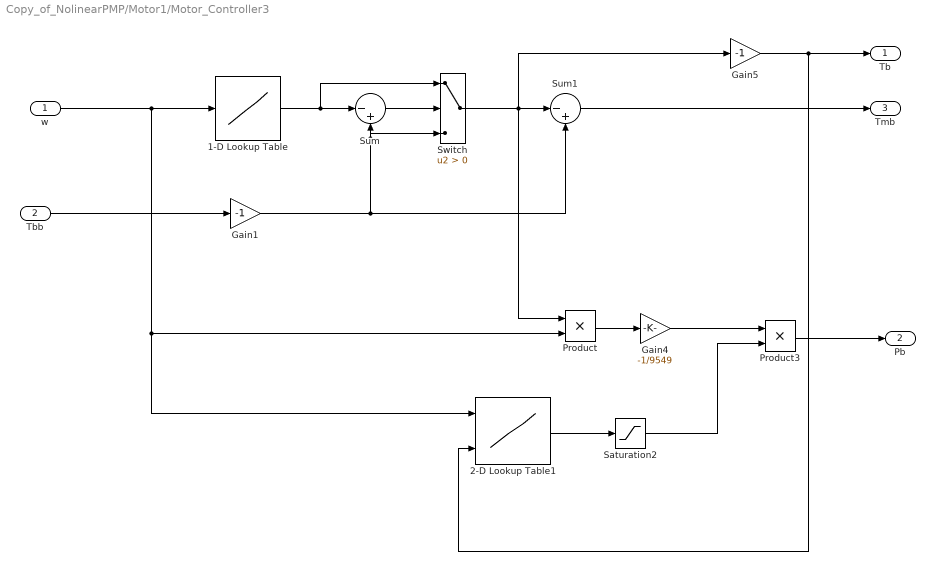
== system Copy_of_NolinearPMP/Motor1/Motor_Controller3 ==
  w : Inport
  Tbb : Inport  Port=2
  1-D Lookup Table : Lookup_n-D  NumberOfTableDimensions=1  BreakpointsForDimension1=motor_nt(:,1)  Table=motor_nt(:,2)*0.6  InternalRulePriority=Speed  RndMeth=Simplest  InputSameDT=on
  2-D Lookup Table1 : Lookup_n-D  BreakpointsForDimension1=0:500:4500  BreakpointsForDimension2=-850:50:850  Table=eff_m  InternalRulePriority=Speed  RndMeth=Simplest  InputSameDT=on
  Gain1 : Gain  Gain=-1
  Gain4 : Gain  Gain=-1/9549
  Gain5 : Gain  Gain=-1
  Product : Product  RndMeth=Zero
  Product3 : Product  RndMeth=Zero
  Saturation2 : Saturate  UpperLimit=1  LowerLimit=0.1
  Sum : Sum  Inputs=|-+
  Sum1 : Sum  Inputs=|-+
  Switch : Switch  Criteria=u2 > Threshold
  Tb : Outport
  Pb : Outport  Port=2
  Tmb : Outport  Port=3
  wires:
  Product/1 -> Gain4/1
  2-D Lookup Table1/1 -> Saturation2/1
  Gain4/1 -> Product3/1
  Tbb/1 -> Gain1/1
  Product3/1 -> Pb/1
  w/1 -> 2-D Lookup Table1/1, Product/2, 1-D Lookup Table/1
  Gain5/1 -> 2-D Lookup Table1/2, Tb/1
  Sum/1 -> Switch/2
  Switch/1 -> Gain5/1, Product/1, Sum1/1
  1-D Lookup Table/1 -> Switch/1, Sum/1
  Gain1/1 -> Sum1/2, Switch/3, Sum/2
  Sum1/1 -> Tmb/1
  Saturation2/1 -> Product3/2

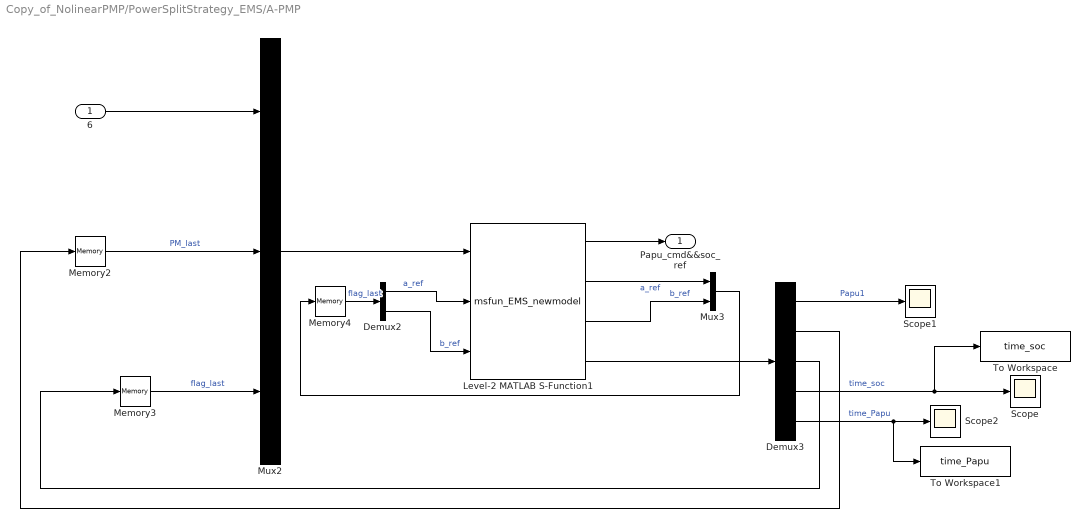
== system Copy_of_NolinearPMP/PowerSplitStrategy_EMS/A-PMP ==
  6 : Inport
  Demux2 : Demux  Outputs=2
  Demux3 : Demux  Outputs=5
  Level-2 MATLAB S-Function1 : M-S-Function  FunctionName=msfun_EMS_newmodel  Parameters=alph_cyc,s,t_cyc,v_cyc,trafficspeed,ess_soc,ess_voc,ess_ro,Np,Ns,Qmax,p2
  Memory2 : Memory  InheritSampleTime=on
  Memory3 : Memory  InheritSampleTime=on
  Memory4 : Memory  InheritSampleTime=on
  Mux2 : Mux  Inputs=3
  Mux3 : Mux  Inputs=2
  Scope : Scope
  Scope1 : Scope
  Scope2 : Scope
  To Workspace : ToWorkspace  VariableName=time_soc  SampleTime=-1
  To Workspace1 : ToWorkspace  VariableName=time_Papu  SampleTime=-1
  Papu_cmd&&soc_ref : Outport
  wires:
  Level-2 MATLAB S-Function1/4 -> Demux3/1
  Memory2/1 -> Mux2/2  "PM_last"
  Demux3/3 -> Memory3/1
  Demux3/2 -> Memory2/1
  Level-2 MATLAB S-Function1/3 -> Mux3/2  "b_ref"
  Level-2 MATLAB S-Function1/2 -> Mux3/1  "a_ref"
  Memory4/1 -> Demux2/1  "flag_last"
  Mux3/1 -> Memory4/1
  Mux2/1 -> Level-2 MATLAB S-Function1/1
  Demux3/1 -> Scope1/1  "Papu1"
  Demux2/1 -> Level-2 MATLAB S-Function1/2  "a_ref"
  Demux2/2 -> Level-2 MATLAB S-Function1/3  "b_ref"
  Memory3/1 -> Mux2/3  "flag_last"
  Level-2 MATLAB S-Function1/1 -> Papu_cmd&&soc_ref/1
  6/1 -> Mux2/1
  Demux3/4 -> To Workspace/1, Scope/1  "time_soc"
  Demux3/5 -> To Workspace1/1, Scope2/1  "time_Papu"

== system Copy_of_NolinearPMP/PowerSplitStrategy_EMS/N-PMP ==
  11INPUT : Inport
  Demux1 : Demux  Outputs=2
  Demux2 : Demux
  Level-2 MATLAB S-Function : M-S-Function  FunctionName=msfun_EMS_PMP  Parameters=meanspeed_record,meangrade,ratio,PM,Qnom,regR,ess_soc,ess_voc,ess_ro,Ns,Np,K,p2,Pdmd_distribution,distance_edge
  Memory1 : Memory  InheritSampleTime=on
  Mux1 : Mux  Inputs=2
  Out1 : Outport
  Out2 : Outport  Port=2
  Out3 : Outport  Port=3  VectorParamsAs1DForOutWhenUnconnected=off
  CDR : Outport  Port=4  VectorParamsAs1DForOutWhenUnconnected=off
  flag : Outport  Port=5  VectorParamsAs1DForOutWhenUnconnected=off
  CDRMethod : Outport  Port=6  VectorParamsAs1DForOutWhenUnconnected=off
  wires:
  Demux1/1 -> Level-2 MATLAB S-Function/2  "s_ref_last"
  Level-2 MATLAB S-Function/2 -> Mux1/1  "s_ref"
  Demux1/2 -> Level-2 MATLAB S-Function/3  "SOC_ref_last"
  Mux1/1 -> Memory1/1
  Memory1/1 -> Demux1/1
  Level-2 MATLAB S-Function/3 -> Mux1/2  "SOC_ref"
  Level-2 MATLAB S-Function/1 -> Demux2/1
  11INPUT/1 -> Level-2 MATLAB S-Function/1
  Demux2/2 -> Out2/1  "soc_ref"
  Demux2/1 -> Out1/1  "Papu_cmd"
  Demux2/3 -> Out3/1  "PMcon"
  Level-2 MATLAB S-Function/4 -> CDR/1
  Demux2/4 -> flag/1
  Level-2 MATLAB S-Function/5 -> CDRMethod/1

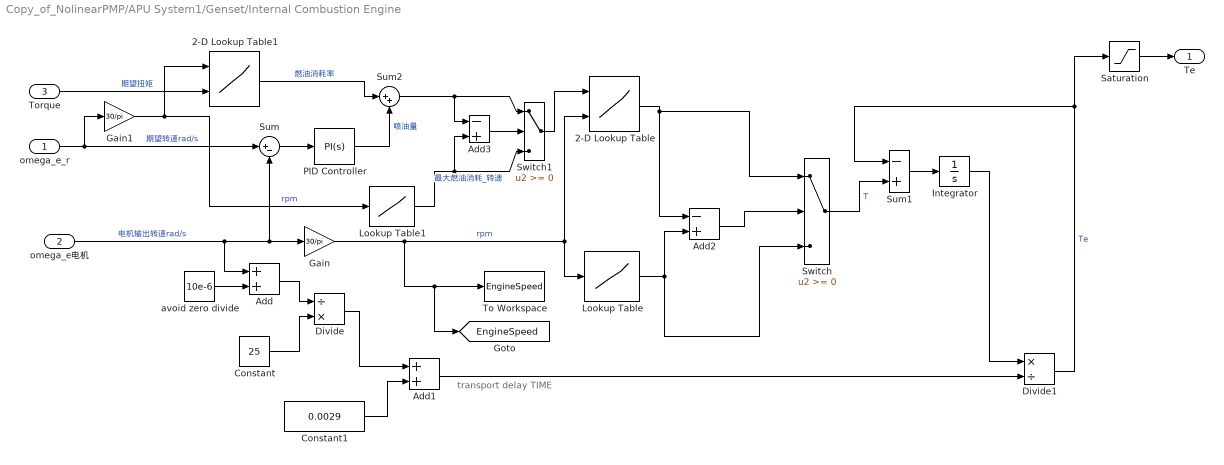
== system Copy_of_NolinearPMP/APU System1/Genset/Internal Combustion Engine ==
  note: transport delay TIME
  omega_e_r : Inport
  omega_e电机 : Inport  Port=2
  Torque : Inport  Port=3
  2-D Lookup Table : Lookup_n-D  BreakpointsForDimension1=0:0.1:5  BreakpointsForDimension2=1000:250:3000  Table=BrakeTorque'  InputSameDT=on
  2-D Lookup Table1 : Lookup_n-D  BreakpointsForDimension1=1000:250:3000  BreakpointsForDimension2=0:5:275  Table=fuelrate  InputSameDT=on
  Add : Sum
  Add1 : Sum
  Add2 : Sum  Inputs=-+
  Add3 : Sum  Inputs=-+
  Constant : Constant  Value=25
  Constant1 : Constant  Value=0.0029
  Divide : Product  Inputs=/*
  Divide1 : Product  Inputs=*/
  Gain : Gain  Gain=30/pi
  Gain1 : Gain  Gain=30/pi
  Integrator : Integrator
  Lookup Table : Lookup  InputValues=[850,1000,1250,1500,1750,2000,2250,2500,2750,3000,3250,3500,3750,4000]  Table=[195,195,195,195.9,244.1,270.2,272.7,269.1,266.6,261.5,257.7,242.9,229.9,221.4]
  Lookup Table1 : Lookup  InputValues=[1000,1250,1500,1750,2000,2250,2500,2750,3000]  Table=MaxFuelRate
  PID Controller : simulink/Continuous/PID Controller  Controller=PI  Form=Parallel  TimeDomain=Continuous-time  SampleTime=-1  IntegratorMethod=Forward Euler  FilterMethod=Forward Euler  ControllerParametersSource=internal  P=0.1  I=0.2  D=0  UseFilter=on  N=100  TunerSelectOption=Transfer Function Based (PID Tuner App)  InitialConditionSource=internal  InitialConditionForIntegrator=0  InitialConditionForFilter=0  DifferentiatorICPrevScaledInput=0  ExternalReset=none  TrackingMode=off  Kt=1  LimitOutput=off  UpperSaturationLimit=inf  LowerSaturationLimit=-inf  LinearizeAsGain=on  AntiWindupMode=none  Kb=1  POutMin=[]  POutMax=[]  IOutMin=[]  IOutMax=[]  DOutMin=[]  DOutMax=[]  NOutMin=[]  NOutMax=[]  SumOutMin=[]  SumOutMax=[]  SaturationOutMin=[]  SaturationOutMax=[]  PParamMin=[]  PParamMax=[]  IParamMin=[]  IParamMax=[]  DParamMin=[]  DParamMax=[]  NParamMin=[]  NParamMax=[]  KbParamMin=[]  KbParamMax=[]  KtParamMin=[]  KtParamMax=[]  KbOutMin=[]  KbOutMax=[]  KtOutMin=[]  KtOutMax=[]  IntegratorOutMin=[]  IntegratorOutMax=[]  FilterOutMin=[]  FilterOutMax=[]  SumI1OutMin=[]  SumI1OutMax=[]  SumI2OutMin=[]  SumI2OutMax=[]  SumI3OutMin=[]  SumI3OutMax=[]  SumI4OutMin=[]  SumI4OutMax=[]  SumDOutMin=[]  SumDOutMax=[]  DifferentiatorOutMin=[]  DifferentiatorOutMax=[]  FilterDiffOutCoefMin=[]  FilterDiffOutCoefMax=[]  ReciprocalOutMin=[]  ReciprocalOutMax=[]  SumDenOutMin=[]  SumDenOutMax=[]  SumNumOutMin=[]  SumNumOutMax=[]  DivideOutMin=[]  DivideOutMax=[]  IntegratorContinuousStateAttributes=''  IntegratorStateMustResolveToSignalObject=off  IntegratorRTWStateStorageClass=Auto  FilterContinuousStateAttributes=''  FilterStateMustResolveToSignalObject=off  FilterRTWStateStorageClass=Auto  ParallelPVariant=InternalParameters  IdealPVariant=Disabled  IVariant=InternalParameters  DVariant=Disabled  IntegratorVariant=Continuous  SatVariant=Disabled  AWVariant=Passthrough  PCopyVariant=Disabled  TRVariant=Disabled  FdbkBlocksVariant=Forward  IdealPFdbkVariant=Disabled  SatFdbkVariant=Disabled  DerivativeFilterVariant=Disabled  NVariant=Disabled  NCopyVariant=Disabled_SignalSpec  FilterICVariant=Disabled  IntegratorICVariant=InternalICs  ExternalResetVariant=Disabled  TRSumVariant=Passthrough  SumFdbkVariant=Disabled  SumVariant=Sum_PI
  Saturation : Saturate  UpperLimit=280  LowerLimit=0  LinearizeAsGain=off
  Sum : Sum  Inputs=|+-
  Sum1 : Sum  Inputs=-+
  Sum2 : Sum  Inputs=|++
  Switch : Switch
  Switch1 : Switch
  To Workspace : ToWorkspace  VariableName=EngineSpeed  SampleTime=-1
  avoid zero divide : Constant  Value=10e-6
  Te : Outport
  tag scope: EngineSpeed=global
  wires:
  omega_e电机/1 -> Add/1, Sum/2, Gain/1  "电机输出转速rad/s"
  Sum/1 -> PID Controller/1
  avoid zero divide/1 -> Add/2
  Constant/1 -> Divide/2
  Add/1 -> Divide/1
  Divide/1 -> Add1/1
  Constant1/1 -> Add1/2
  Add1/1 -> Divide1/2
  Integrator/1 -> Divide1/1
  Sum1/1 -> Integrator/1
  2-D Lookup Table/1 -> Add2/1, Switch/1
  Lookup Table/1 -> Add2/2, Switch/3
  Divide1/1 -> Sum1/1, Saturation/1  "Te"
  omega_e_r/1 -> Gain1/1, Sum/1  "期望转速rad/s"
  Gain/1 -> Lookup Table/1, 2-D Lookup Table/2, To Workspace/1, [EngineSpeed]  "rpm"
  Add2/1 -> Switch/2
  Switch/1 -> Sum1/2  "T"
  2-D Lookup Table1/1 -> Sum2/1  "燃油消耗率"
  PID Controller/1 -> Sum2/2  "喷油量"
  Sum2/1 -> Add3/1, Switch1/1
  Torque/1 -> 2-D Lookup Table1/2  "期望扭矩"
  Gain1/1 -> 2-D Lookup Table1/1, Lookup Table1/1  "rpm"
  Lookup Table1/1 -> Add3/2, Switch1/3  "最大燃油消耗_转速"
  Add3/1 -> Switch1/2
  Switch1/1 -> 2-D Lookup Table/1
  Saturation/1 -> Te/1

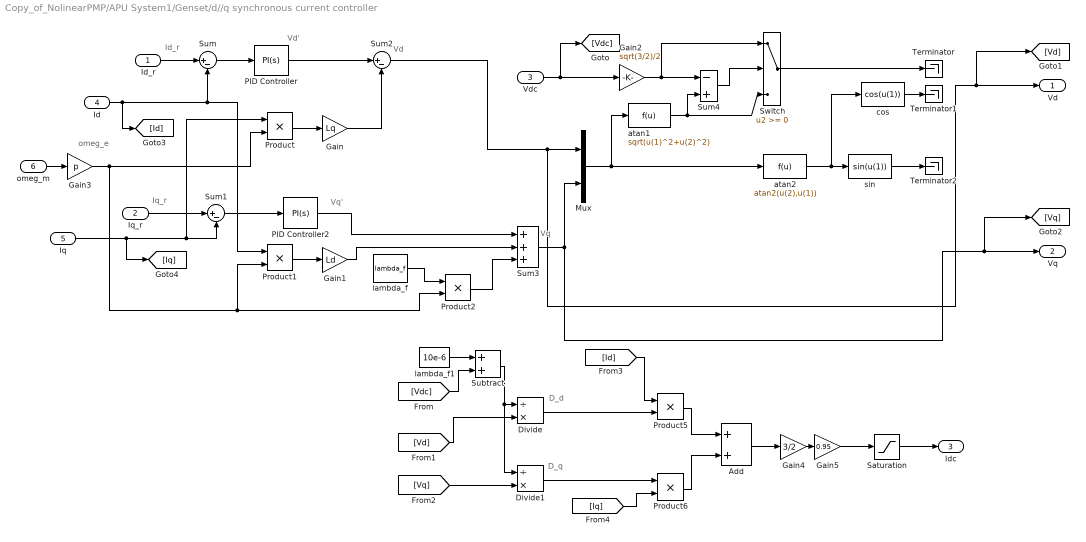
== system Copy_of_NolinearPMP/APU System1/Genset/d//q synchronous current controller ==
  note: Id_r
  note: Iq_r
  note: Vd'
  note: Vq'
  note: Vd
  note: Vq
  note: omeg_e
  note: D_d
  note: D_q
  Id_r : Inport
  Iq_r : Inport  Port=2
  Vdc : Inport  Port=3
  Id : Inport  Port=4
  Iq : Inport  Port=5
  omeg_m : Inport  Port=6
  Add : Sum
  Divide : Product  Inputs=/*
  Divide1 : Product  Inputs=/*
  Gain : Gain  Gain=Lq
  Gain1 : Gain  Gain=Ld
  Gain2 : Gain  Gain=sqrt(3/2)/2
  Gain3 : Gain  Gain=p
  Gain4 : Gain  Gain=3/2
  Gain5 : Gain  Gain=0.95
  Mux : Mux  Inputs=2
  PID Controller : simulink/Continuous/PID Controller  Controller=PI  Form=Parallel  TimeDomain=Continuous-time  SampleTime=-1  IntegratorMethod=Forward Euler  FilterMethod=Forward Euler  ControllerParametersSource=internal  P=0.003  I=0.01  D=0  UseFilter=on  N=100  TunerSelectOption=Transfer Function Based (PID Tuner App)  InitialConditionSource=internal  InitialConditionForIntegrator=0  InitialConditionForFilter=0  DifferentiatorICPrevScaledInput=0  ExternalReset=none  TrackingMode=off  Kt=1  LimitOutput=off  UpperSaturationLimit=inf  LowerSaturationLimit=-inf  LinearizeAsGain=on  AntiWindupMode=none  Kb=1  POutMin=[]  POutMax=[]  IOutMin=[]  IOutMax=[]  DOutMin=[]  DOutMax=[]  NOutMin=[]  NOutMax=[]  SumOutMin=[]  SumOutMax=[]  SaturationOutMin=[]  SaturationOutMax=[]  PParamMin=[]  PParamMax=[]  IParamMin=[]  IParamMax=[]  DParamMin=[]  DParamMax=[]  NParamMin=[]  NParamMax=[]  KbParamMin=[]  KbParamMax=[]  KtParamMin=[]  KtParamMax=[]  KbOutMin=[]  KbOutMax=[]  KtOutMin=[]  KtOutMax=[]  IntegratorOutMin=[]  IntegratorOutMax=[]  FilterOutMin=[]  FilterOutMax=[]  SumI1OutMin=[]  SumI1OutMax=[]  SumI2OutMin=[]  SumI2OutMax=[]  SumI3OutMin=[]  SumI3OutMax=[]  SumI4OutMin=[]  SumI4OutMax=[]  SumDOutMin=[]  SumDOutMax=[]  DifferentiatorOutMin=[]  DifferentiatorOutMax=[]  FilterDiffOutCoefMin=[]  FilterDiffOutCoefMax=[]  ReciprocalOutMin=[]  ReciprocalOutMax=[]  SumDenOutMin=[]  SumDenOutMax=[]  SumNumOutMin=[]  SumNumOutMax=[]  DivideOutMin=[]  DivideOutMax=[]  IntegratorContinuousStateAttributes=''  IntegratorStateMustResolveToSignalObject=off  IntegratorRTWStateStorageClass=Auto  FilterContinuousStateAttributes=''  FilterStateMustResolveToSignalObject=off  FilterRTWStateStorageClass=Auto  ParallelPVariant=InternalParameters  IdealPVariant=Disabled  IVariant=InternalParameters  DVariant=Disabled  IntegratorVariant=Continuous  SatVariant=Disabled  AWVariant=Passthrough  PCopyVariant=Disabled  TRVariant=Disabled  FdbkBlocksVariant=Forward  IdealPFdbkVariant=Disabled  SatFdbkVariant=Disabled  DerivativeFilterVariant=Disabled  NVariant=Disabled  NCopyVariant=Disabled_SignalSpec  FilterICVariant=Disabled  IntegratorICVariant=InternalICs  ExternalResetVariant=Disabled  TRSumVariant=Passthrough  SumFdbkVariant=Disabled  SumVariant=Sum_PI
  PID Controller2 : simulink/Continuous/PID Controller  Controller=PI  Form=Parallel  TimeDomain=Continuous-time  SampleTime=-1  IntegratorMethod=Forward Euler  FilterMethod=Forward Euler  ControllerParametersSource=internal  P=0.3  I=0.3  D=0  UseFilter=on  N=100  TunerSelectOption=Transfer Function Based (PID Tuner App)  InitialConditionSource=internal  InitialConditionForIntegrator=0  InitialConditionForFilter=0  DifferentiatorICPrevScaledInput=0  ExternalReset=none  TrackingMode=off  Kt=1  LimitOutput=off  UpperSaturationLimit=inf  LowerSaturationLimit=-inf  LinearizeAsGain=on  AntiWindupMode=none  Kb=1  POutMin=[]  POutMax=[]  IOutMin=[]  IOutMax=[]  DOutMin=[]  DOutMax=[]  NOutMin=[]  NOutMax=[]  SumOutMin=[]  SumOutMax=[]  SaturationOutMin=[]  SaturationOutMax=[]  PParamMin=[]  PParamMax=[]  IParamMin=[]  IParamMax=[]  DParamMin=[]  DParamMax=[]  NParamMin=[]  NParamMax=[]  KbParamMin=[]  KbParamMax=[]  KtParamMin=[]  KtParamMax=[]  KbOutMin=[]  KbOutMax=[]  KtOutMin=[]  KtOutMax=[]  IntegratorOutMin=[]  IntegratorOutMax=[]  FilterOutMin=[]  FilterOutMax=[]  SumI1OutMin=[]  SumI1OutMax=[]  SumI2OutMin=[]  SumI2OutMax=[]  SumI3OutMin=[]  SumI3OutMax=[]  SumI4OutMin=[]  SumI4OutMax=[]  SumDOutMin=[]  SumDOutMax=[]  DifferentiatorOutMin=[]  DifferentiatorOutMax=[]  FilterDiffOutCoefMin=[]  FilterDiffOutCoefMax=[]  ReciprocalOutMin=[]  ReciprocalOutMax=[]  SumDenOutMin=[]  SumDenOutMax=[]  SumNumOutMin=[]  SumNumOutMax=[]  DivideOutMin=[]  DivideOutMax=[]  IntegratorContinuousStateAttributes=''  IntegratorStateMustResolveToSignalObject=off  IntegratorRTWStateStorageClass=Auto  FilterContinuousStateAttributes=''  FilterStateMustResolveToSignalObject=off  FilterRTWStateStorageClass=Auto  ParallelPVariant=InternalParameters  IdealPVariant=Disabled  IVariant=InternalParameters  DVariant=Disabled  IntegratorVariant=Continuous  SatVariant=Disabled  AWVariant=Passthrough  PCopyVariant=Disabled  TRVariant=Disabled  FdbkBlocksVariant=Forward  IdealPFdbkVariant=Disabled  SatFdbkVariant=Disabled  DerivativeFilterVariant=Disabled  NVariant=Disabled  NCopyVariant=Disabled_SignalSpec  FilterICVariant=Disabled  IntegratorICVariant=InternalICs  ExternalResetVariant=Disabled  TRSumVariant=Passthrough  SumFdbkVariant=Disabled  SumVariant=Sum_PI
  Product{,1..2,5..6} (5 alike) : Product  RndMeth=Zero
  Saturation : Saturate  UpperLimit=180  LowerLimit=0
  Subtract : Sum
  Sum : Sum  Inputs=|+-
  Sum1 : Sum  Inputs=|+-
  Sum2 : Sum  Inputs=|+-
  Sum3 : Sum  Inputs=+++
  Sum4 : Sum  Inputs=-+
  Switch : Switch
  Terminator : Terminator
  Terminator1 : Terminator
  Terminator2 : Terminator
  atan1 : Fcn  Expr=sqrt(u(1)^2+u(2)^2)
  atan2 : Fcn  Expr=atan2(u(2),u(1))
  cos : Fcn  Expr=cos(u(1))
  lambda_f : Constant  Value=lambda_f
  lambda_f1 : Constant  Value=10e-6
  sin : Fcn  Expr=sin(u(1))
  Vd : Outport
  Vq : Outport  Port=2
  Idc : Outport  Port=3
  wires:
  Id_r/1 -> Sum/1
  Id/1 -> Sum/2, Product1/1, [Id]
  Sum/1 -> PID Controller/1
  Iq_r/1 -> Sum1/1
  Sum1/1 -> PID Controller2/1
  PID Controller/1 -> Sum2/1
  Product/1 -> Gain/1
  Gain/1 -> Sum2/2
  Sum2/1 -> Mux/1, Vd/1, [Vd]
  Product1/1 -> Gain1/1
  Gain1/1 -> Sum3/2
  Product2/1 -> Sum3/3
  lambda_f/1 -> Product2/1
  Sum3/1 -> Mux/2, Vq/1, [Vq]
  Mux/1 -> atan1/1, atan2/1
  atan2/1 -> cos/1, sin/1
  cos/1 -> Terminator1/1
  sin/1 -> Terminator2/1
  Iq/1 -> Sum1/2, Product/1, [Iq]
  Gain3/1 -> Product/2, Product1/2, Product2/2
  omeg_m/1 -> Gain3/1
  Vdc/1 -> [Vdc], Gain2/1
  atan1/1 -> Sum4/2, Switch/3
  Sum4/1 -> Switch/2
  Switch/1 -> Terminator/1
  PID Controller2/1 -> Sum3/1
  [Vdc] -> Subtract/2
  [Vd] -> Divide/2
  [Vq] -> Divide1/2
  [Id] -> Product5/1
  Divide/1 -> Product5/2
  Divide1/1 -> Product6/1
  [Iq] -> Product6/2
  Product5/1 -> Add/1
  Product6/1 -> Add/2
  Add/1 -> Gain4/1
  Gain4/1 -> Gain5/1
  lambda_f1/1 -> Subtract/1
  Subtract/1 -> Divide1/1, Divide/1
  Saturation/1 -> Idc/1
  Gain5/1 -> Saturation/1
  Gain2/1 -> Sum4/1, Switch/1

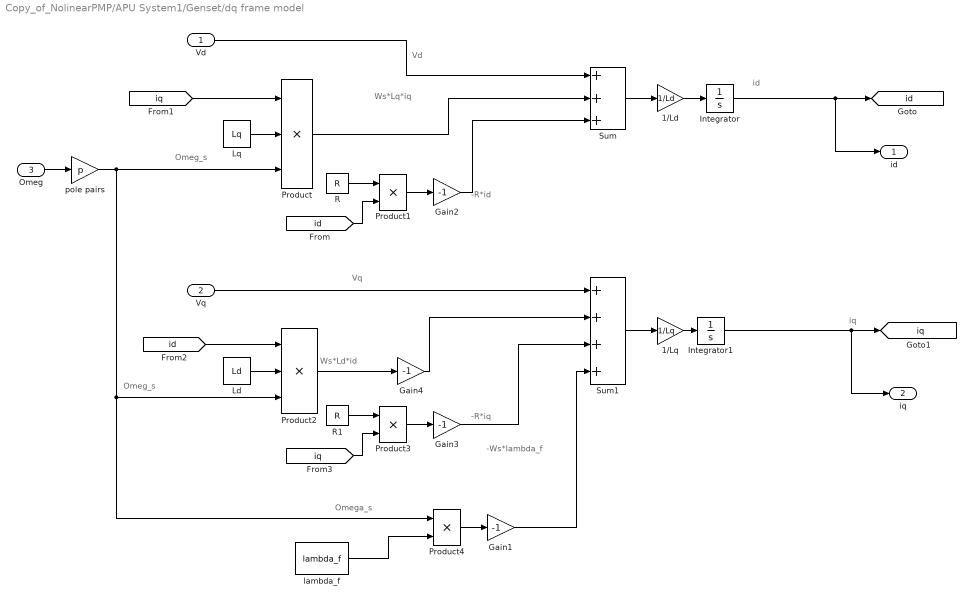
== system Copy_of_NolinearPMP/APU System1/Genset/dq frame model  ==
  note: Omeg_s
  note: Vd
  note: Ws*Lq*iq
  note: -R*id
  note: id
  note: Vq
  note: Ws*Ld*id
  note: -R*iq
  note: Omeg_s
  note: Omega_s
  note: -Ws*lambda_f
  note: iq
  Vd : Inport
  Vq : Inport  Port=2
  Omeg : Inport  Port=3
  1/Ld : Gain  Gain=1/Ld
  1/Lq : Gain  Gain=1/Lq
  Gain{1..4} (4 alike) : Gain  Gain=-1
  Integrator : Integrator
  Integrator1 : Integrator  LimitOutput=on  UpperSaturationLimit=2/3/(p*lambda_f)*280  LowerSaturationLimit=0
  Ld : Constant  Value=Ld
  Lq : Constant  Value=Lq
  Product : Product  Inputs=3  RndMeth=Zero
  Product1 : Product  RndMeth=Zero
  Product2 : Product  Inputs=3  RndMeth=Zero
  Product3 : Product  RndMeth=Zero
  Product4 : Product  RndMeth=Zero
  R : Constant  Value=R
  R1 : Constant  Value=R
  Sum : Sum  Inputs=+++
  Sum1 : Sum  Inputs=++++
  lambda_f : Constant  Value=lambda_f
  pole pairs : Gain  Gain=p
  id : Outport
  iq : Outport  Port=2
  tag scope: id=global, iq=global
  wires:
  Omeg/1 -> pole pairs/1
  pole pairs/1 -> Product4/1, Product2/3, Product/3
  Lq/1 -> Product/2
  Product/1 -> Sum/2
  R/1 -> Product1/1
  Sum/1 -> 1/Ld/1
  1/Ld/1 -> Integrator/1
  Integrator/1 -> id/1, [id]
  [id] -> Product1/2
  [iq] -> Product/1
  Ld/1 -> Product2/2
  [id] -> Product2/1
  Product1/1 -> Gain2/1
  Gain2/1 -> Sum/3
  R1/1 -> Product3/1
  [iq] -> Product3/2
  Product3/1 -> Gain3/1
  Gain3/1 -> Sum1/3
  Product2/1 -> Gain4/1
  Gain4/1 -> Sum1/2
  lambda_f/1 -> Product4/2
  Sum1/1 -> 1/Lq/1
  1/Lq/1 -> Integrator1/1
  Integrator1/1 -> [iq], iq/1
  Vd/1 -> Sum/1
  Vq/1 -> Sum1/1
  Product4/1 -> Gain1/1
  Gain1/1 -> Sum1/4

== system Copy_of_NolinearPMP/APU System1/Genset/mechanical part ==
  note: Te
  note: alpha
  id : Inport
  iq : Inport  Port=2
  Teng : Inport  Port=3
  Constant : Constant
  Gain : Gain  Gain=lambda_f
  Gain1 : Gain  Gain=Ld-Lq
  Integrator : Integrator  InitialCondition=1000*pi/30
  Jg : Gain  Gain=1/(Je+Jg)
  Jg1 : Gain  Gain=3*p/2
  Product : Product  RndMeth=Zero
  Saturation : Saturate  UpperLimit=3200*pi/30  LowerLimit=750*pi/30
  Sum : Sum
  Sum2 : Sum  Inputs=-+-
  omeg : Outport
  wires:
  iq/1 -> Product/2, Gain/1
  id/1 -> Product/1
  Gain/1 -> Sum/2
  Product/1 -> Gain1/1
  Gain1/1 -> Sum/1
  Sum/1 -> Jg1/1
  Teng/1 -> Sum2/2
  Sum2/1 -> Jg/1
  Jg/1 -> Integrator/1
  Jg1/1 -> Sum2/1
  Integrator/1 -> Saturation/1
  Saturation/1 -> omeg/1
  Constant/1 -> Sum2/3

== system Copy_of_NolinearPMP/Driver1/Driver/LPF00 ==
  u1 : Inport
  Constant1 : Constant  Value=0.03  SampleTime=-1
  Divide1 : Product  Inputs=/
  Integrator1 : Integrator
  Product1 : Product  RndMeth=Zero
  Sum1 : Sum  Inputs=|+-
  y1 : Outport
  wires:
  u1/1 -> Sum1/1
  Product1/1 -> Integrator1/1
  Divide1/1 -> Product1/1
  Integrator1/1 -> y1/1, Sum1/2
  Constant1/1 -> Divide1/1
  Sum1/1 -> Product1/2

== stateflow chart Copy_of_NolinearPMP/Control Strategy ==
  state Controller
    state GearShifting [parallel]
      settings: executionOrder=1
      state first
        entry:
        GearCmd = 1;
      state second
        entry:
        GearCmd = 2;
      (default) -> first
      first -> second : [Velocity>20]
      second -> first : [Velocity<15]
    state PedelInterp [parallel]
      settings: executionOrder=2
      state Drving
        du: Td = Acc*8000;Tb = 0;
      state Braking
        du:Td = 0; Tb = Bra*-1800;
      (junction 17) -> Drving [order 1] : [Bra<=0]
      Braking -> Drving : [Acc>0]
      Drving -> Braking : [Bra>0]
      (default) -> (junction 17)
      (junction 17) -> Braking [order 2] : [Bra>0]
  (default) -> Controller
  data: Acc input [0..1]; Bra input [0..1]; Velocity input; GearCmd output double; Td output double; Tb output double; s local double; ss local double
  events: Sampling input RISING_EDGE_EVENT
